simulink model "gmStateSpaceHDL_buck_convert_test1_REFERENCE"  (R2025a)
settings: Solver=FixedStepDiscrete  StartTime=0.0  StopTime=0.005  RelTol=1e-3  AbsTol=1e-3
InitFcn:
  | load('C:\Users\bensa\Desktop\PI3_FPGA_BuckConverter\sschdl\buck_convert_test1\stateSpaceParameters.mat');
model workspace (MAT data in the model file):
  NoaFutureIOMap{1}.PortName = 'rst'
  NoaFutureIOMap{1}.PortType = 'Inport'
  NoaFutureIOMap{1}.DataType = 'uint32'
  NoaFutureIOMap{1}.IOInterface = 'AXI4-Lite'
  NoaFutureIOMap{1}.IOInterfaceMapping = 'x"100"'
  NoaFutureIOMap{2}.PortName = 'duty'
  NoaFutureIOMap{2}.PortType = 'Inport'
  NoaFutureIOMap{2}.DataType = 'uint32'
  NoaFutureIOMap{2}.IOInterface = 'AXI4-Lite'
  NoaFutureIOMap{2}.IOInterfaceMapping = 'x"104"'
  NoaFutureIOMap{3}.PortName = 'freq'
  NoaFutureIOMap{3}.PortType = 'Inport'
  NoaFutureIOMap{3}.DataType = 'uint32'
  NoaFutureIOMap{3}.IOInterface = 'AXI4-Lite'
  NoaFutureIOMap{3}.IOInterfaceMapping = 'x"108"'
  NoaFutureIOMap{4}.PortName = 'en'
  NoaFutureIOMap{4}.PortType = 'Inport'
  NoaFutureIOMap{4}.DataType = 'uint32'
  NoaFutureIOMap{4}.IOInterface = 'AXI4-Lite'
  NoaFutureIOMap{4}.IOInterfaceMapping = 'x"10C"'
  NoaFutureIOMap{5}.PortName = 'vout'
  NoaFutureIOMap{5}.PortType = 'Outport'
  NoaFutureIOMap{5}.DataType = 'single'
  NoaFutureIOMap{5}.IOInterface = 'DAQ Channel 0 [0:31]'
  NoaFutureIOMap{5}.IOInterfaceMapping = '[0:31]'
  NoaFutureIOMap{6}.PortName = 'vin'
  NoaFutureIOMap{6}.PortType = 'Outport'
  NoaFutureIOMap{6}.DataType = 'single'
  NoaFutureIOMap{6}.IOInterface = 'DAQ Channel 1 [0:31]'
  NoaFutureIOMap{6}.IOInterfaceMapping = '[0:31]'
  NoaFutureIOMap{7}.PortName = 'vout_a'
  NoaFutureIOMap{7}.PortType = 'Outport'
  NoaFutureIOMap{7}.DataType = 'sfix32_En27'
  NoaFutureIOMap{7}.IOInterface = 'Analog Output 0 [0:31]'
  NoaFutureIOMap{7}.IOInterfaceMapping = '[0:31]'
  NoaFutureIOMap{7}.NoaBlockParameters.SignalMin = '0'
  NoaFutureIOMap{7}.NoaBlockParameters.SignalMax = '12'
  NoaFutureIOMap{7}.NoaBlockParameters.VoltageMin = '0'
  NoaFutureIOMap{7}.NoaBlockParameters.VoltageMax = '4'
  NoaFutureIOMap{7}.NoaBlockParameters.LUT_Signals = '[0          1.2          2.4          3.6          4.8            6          7.2          8.4          9.6         10.8           12]'
  NoaFutureIOMap{7}.NoaBlockParameters.LUT_Values = '[0         0.4         0.8         1.2         1.6           2         2.4         2.8         3.2         3.6           4]'
values from neighbouring files (symbols this model uses):
  stateSpaceParameters_1 =     [stateSpaceParameters.mat]
libraries: hdlsllib x4, hdlssclib x4, library_AnalogOut x1, simulink x1
CloseFcn:
  | clear stateSpaceParameters_1
settings Model: DataTypeOverride=Off  Creator=bensa  LastModifiedBy=bensa
settings SolverCC: AutoScaleAbsTol=off  AlgebraicLoopSolver=TrustRegion  MaxZcPerStep=1.0
settings OptimizationCC: BlockReduction=off  ConditionallyExecuteInputs=off  DefaultParameterBehavior=Inlined  InheritOutputTypeSmallerThanSingle=on
settings DebuggingCC: AlgebraicLoopMsg=error  ArtificialAlgebraicLoopMsg=error  SingleTaskRateTransMsg=error  UnconnectedInputMsg=warning  UnconnectedOutputMsg=warning  UnconnectedLineMsg=warning  SymbolicDimsDataTypeCodeGenerationDiagnostic=none
settings HardwareCC: ProdBitPerPointer=32.0  ProdBitPerSizeT=32.0  ProdBitPerPtrDiffT=32.0  ProdLargestAtomicFloat=None  ProdIntDivRoundTo=Undefined  ProdEndianess=Unspecified  ProdWordSize=32.0  ProdHWDeviceType=ASIC/FPGA->ASIC/FPGA  TargetBitPerPointer=64.0  TargetBitPerSizeT=64.0  TargetBitPerPtrDiffT=64.0  TargetLongLongMode=on  TargetIntDivRoundTo=Zero  TargetEndianess=LittleEndian  TargetWordSize=64.0  TargetHWDeviceType=Custom Processor->MATLAB Host Computer  ProdEqTarget=off
settings ModelReferenceCC: EnableRefExpFcnMdlSchedulingChecks=on
settings SFSimCC: CustomCodeUndefinedFunction=UseInterfaceOnly
settings RTWCC: GPUComputeCapability=3.5  DLArmComputeVersion=19.05
settings SimscapeCC: SimscapeLogType=all  SimscapeLogSimulationStatistics=on  SimscapeLogDataHistory=10000.0

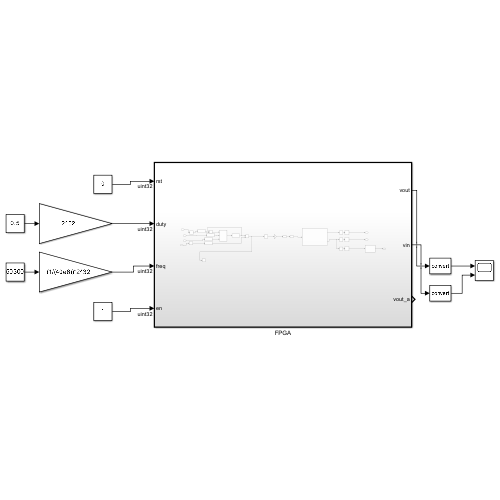
[thumbnail: Simulink's stored preview of the top-level diagram]
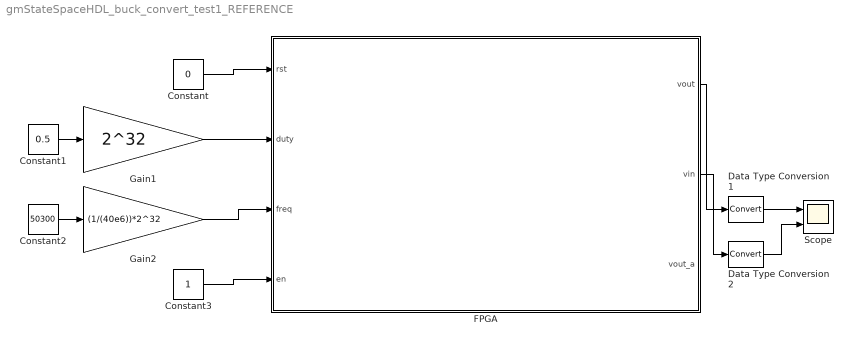
== system gmStateSpaceHDL_buck_convert_test1_REFERENCE ==
  Constant : Constant  Value=0  OutDataTypeStr=uint32  SampleTime=25e-9
  Constant1 : Constant  Value=0.5  OutDataTypeStr=double  SampleTime=25e-9
  Constant2 : Constant  Value=50300  SampleTime=25e-9
  Constant3 : Constant  OutDataTypeStr=uint32  SampleTime=25e-9
  Data Type Conversion1 : DataTypeConversion  RndMeth=Nearest  SaturateOnIntegerOverflow=off  LockScale=on
  Data Type Conversion2 : DataTypeConversion  RndMeth=Nearest  SaturateOnIntegerOverflow=off  LockScale=on
  FPGA : Subsystem  TreatAsAtomicUnit=on
  Gain1 : Gain  Gain=2^32  OutDataTypeStr=uint32
  Gain2 : Gain  Gain=(1/(40e6))*2^32  OutDataTypeStr=uint32
  Scope : Scope  NumInputPorts=2
      settings: ActiveDisplayYMinimum=-1.4999999999999996  ActiveDisplayYMaximum=13.5
  wires:
  Data Type Conversion1/1 -> Scope/1
  Data Type Conversion2/1 -> Scope/2
  FPGA/1(vout) -> Data Type Conversion1/1
  FPGA/2(vin) -> Data Type Conversion2/1
  Constant1/1 -> Gain1/1
  Constant/1 -> FPGA/1(rst)
  Constant2/1 -> Gain2/1
  Gain1/1 -> FPGA/2(duty)
  Gain2/1 -> FPGA/3(freq)
  Constant3/1 -> FPGA/4(en)

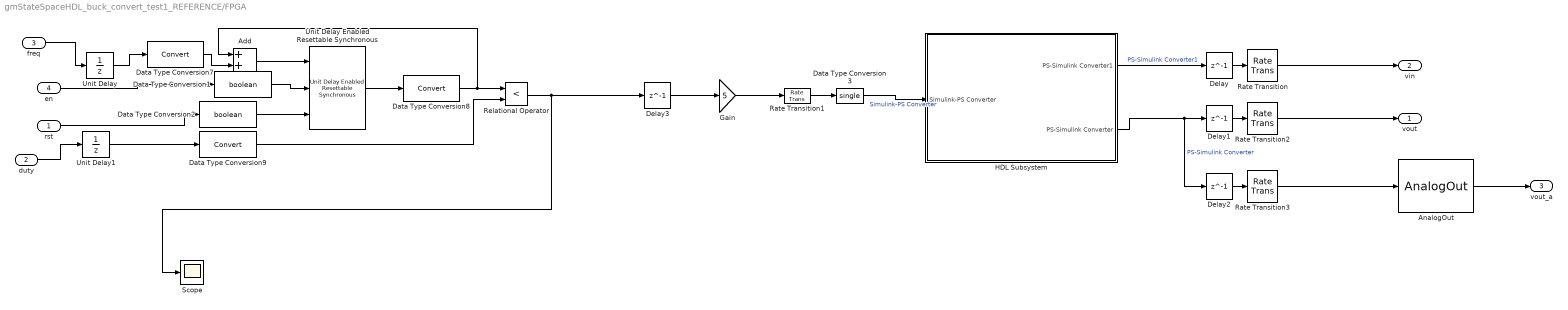
== system gmStateSpaceHDL_buck_convert_test1_REFERENCE/FPGA ==
  rst : Inport  OutDataTypeStr=uint32
  duty : Inport  Port=2  OutDataTypeStr=uint32
  freq : Inport  Port=3  OutDataTypeStr=uint32
  en : Inport  Port=4  OutDataTypeStr=uint32
  Add : Sum  OutDataTypeStr=uint32  AccumDataTypeStr=uint32
  AnalogOut : library_AnalogOut/AnalogOut  SignalMin=0  SignalMax=12  VoltageMin=0  VoltageMax=4
  Data Type Conversion1 : DataTypeConversion  OutDataTypeStr=boolean  SaturateOnIntegerOverflow=off  RndMeth=Floor
  Data Type Conversion2 : DataTypeConversion  OutDataTypeStr=boolean  SaturateOnIntegerOverflow=off  RndMeth=Floor
  Data Type Conversion3 : DataTypeConversion  OutDataTypeStr=single  RndMeth=Nearest  SaturateOnIntegerOverflow=off
  Data Type Conversion7 : DataTypeConversion  SaturateOnIntegerOverflow=off  RndMeth=Floor
  Data Type Conversion8 : DataTypeConversion  SaturateOnIntegerOverflow=off  RndMeth=Floor
  Data Type Conversion9 : DataTypeConversion  SaturateOnIntegerOverflow=off  RndMeth=Floor
  Delay{,1..3} (4 alike) : Delay  DelayLength=1
  Gain : Gain  Gain=5
  HDL Subsystem : Subsystem
  Rate Transition : RateTransition  OutPortSampleTime=25e-9
  Rate Transition1 : RateTransition  OutPortSampleTime=5e-08
  Rate Transition2 : RateTransition  OutPortSampleTime=25e-9
  Rate Transition3 : RateTransition  OutPortSampleTime=25e-9
  Relational Operator : RelationalOperator  Operator=<  OutDataTypeStr=boolean  RndMeth=Simplest  InputSameDT=off
  Scope : Scope
      settings: ActiveDisplayYMinimum=0.63603790546315564  ActiveDisplayYMaximum=1.1529609907534577
  Unit Delay : UnitDelay  SampleTime=-1  HasFrameUpgradeWarning=on
  Unit Delay Enabled Resettable Synchronous : hdlsllib/Discrete/Unit Delay Enabled Resettable Synchronous  InitialCondition=0.0  SampleTime=-1
  Unit Delay1 : UnitDelay  SampleTime=-1  HasFrameUpgradeWarning=on
  vout : Outport
  vin : Outport  Port=2
  vout_a : Outport  Port=3
  wires:
  HDL Subsystem/2(PS-Simulink Converter) -> Delay2/1, Delay1/1  "PS-Simulink Converter"
  HDL Subsystem/1(PS-Simulink Converter1) -> Delay/1  "PS-Simulink Converter1"
  Rate Transition1/1 -> Data Type Conversion3/1
  Data Type Conversion3/1 -> HDL Subsystem/1(Simulink-PS Converter)  "Simulink-PS Converter"
  Data Type Conversion8/1 -> Add/1, Relational Operator/1
  Add/1 -> Unit Delay Enabled Resettable Synchronous/1
  Unit Delay Enabled Resettable Synchronous/1 -> Data Type Conversion8/1
  Data Type Conversion7/1 -> Add/2
  Data Type Conversion9/1 -> Relational Operator/2
  Unit Delay1/1 -> Data Type Conversion9/1
  Unit Delay/1 -> Data Type Conversion7/1
  Relational Operator/1 -> Scope/1, Delay3/1
  freq/1 -> Unit Delay/1
  duty/1 -> Unit Delay1/1
  rst/1 -> Data Type Conversion2/1
  en/1 -> Data Type Conversion1/1
  Rate Transition/1 -> vin/1
  Rate Transition2/1 -> vout/1
  Delay/1 -> Rate Transition/1
  Delay1/1 -> Rate Transition2/1
  Delay2/1 -> Rate Transition3/1
  Rate Transition3/1 -> AnalogOut/1
  AnalogOut/1 -> vout_a/1
  Data Type Conversion1/1 -> Unit Delay Enabled Resettable Synchronous/2
  Data Type Conversion2/1 -> Unit Delay Enabled Resettable Synchronous/3
  Delay3/1 -> Gain/1
  Gain/1 -> Rate Transition1/1

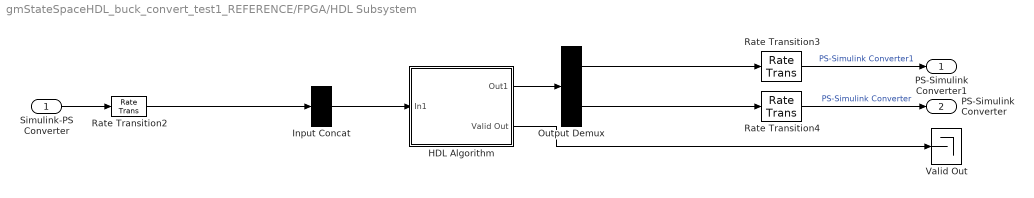
== system gmStateSpaceHDL_buck_convert_test1_REFERENCE/FPGA/HDL Subsystem ==
  Simulink-PS Converter : Inport
  HDL Algorithm : Subsystem
  Input Concat : Concatenate  NumInputs=1
  Output Demux : Demux  Outputs=2
  Rate Transition2 : RateTransition  Integrity=off  OutPortSampleTimeOpt=Multiple of input port sample time  OutPortSampleTimeMultiple=1/2
  Rate Transition3 : RateTransition  OutPortSampleTimeOpt=Multiple of input port sample time  OutPortSampleTimeMultiple=2
  Rate Transition4 : RateTransition  OutPortSampleTimeOpt=Multiple of input port sample time  OutPortSampleTimeMultiple=2
  Valid Out : Terminator
  PS-Simulink Converter1 : Outport
  PS-Simulink Converter : Outport  Port=2
  wires:
  Rate Transition3/1 -> PS-Simulink Converter1/1  "PS-Simulink Converter1"
  Rate Transition2/1 -> Input Concat/1
  HDL Algorithm/1(Out1) -> Output Demux/1
  Input Concat/1 -> HDL Algorithm/1(In1)
  Output Demux/2 -> Rate Transition4/1
  HDL Algorithm/2(Valid Out) -> Valid Out/1
  Output Demux/1 -> Rate Transition3/1
  Rate Transition4/1 -> PS-Simulink Converter/1  "PS-Simulink Converter"
  Simulink-PS Converter/1 -> Rate Transition2/1

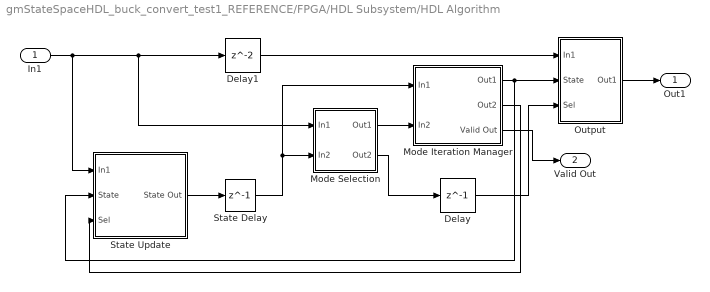
== system gmStateSpaceHDL_buck_convert_test1_REFERENCE/FPGA/HDL Subsystem/HDL Algorithm ==
  In1 : Inport
  Delay : Delay  DelayLength=1
  Delay1 : Delay
  Mode Iteration Manager : Subsystem
  Mode Selection : Subsystem
  Output : Subsystem
  State Delay : Delay  DelayLength=1  InitialCondition=single(stateSpaceParameters_1.X0)
  State Update : Subsystem
  Out1 : Outport  VectorParamsAs1DForOutWhenUnconnected=off
  Valid Out : Outport  Port=2  VectorParamsAs1DForOutWhenUnconnected=off
  wires:
  Mode Iteration Manager/2(Out2) -> State Update/3(Sel)
  In1/1 -> Mode Selection/1(In1), Delay1/1, State Update/1(In1)
  State Update/1(State Out) -> State Delay/1
  Mode Selection/1(Out1) -> Mode Iteration Manager/2(In2)
  Delay1/1 -> Output/1(In1)
  State Delay/1 -> Mode Iteration Manager/1(In1), Mode Selection/2(In2)
  Mode Selection/2(Out2) -> Delay/1
  Mode Iteration Manager/1(Out1) -> State Update/2(State), Output/2(State)
  Mode Iteration Manager/3(Valid Out) -> Valid Out/1
  Delay/1 -> Output/3(Sel)
  Output/1(Out1) -> Out1/1

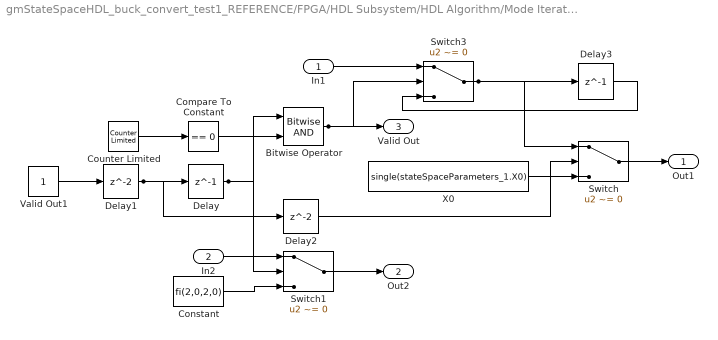
== system gmStateSpaceHDL_buck_convert_test1_REFERENCE/FPGA/HDL Subsystem/HDL Algorithm/Mode Iteration Manager ==
  In1 : Inport  LockScale=on
  In2 : Inport  Port=2  OutDataTypeStr=fixdt(0,2,0)  LockScale=on
  Bitwise Operator : simulink/Logic and Bit Operations/Bitwise Operator  logicop=AND  UseBitMask=off  NumInputPorts=2  BitMask=bin2dec('11011001')  BitMaskRealWorld=Stored Integer
      settings: LibrarySourceBlock=|
      | hdlsllib/Logic and Bit
      | Operations/Bitwise
      | Operator
  Compare To Constant : hdlsllib/Logic and Bit Operations/Compare To Constant  relop===  const=0  OutDataTypeStr=boolean
  Constant : Constant  Value=fi(2,0,2,0)  SampleTime=2.5e-08  LockScale=on
  Counter Limited : hdlsllib/Sources/Counter Limited  uplimit=1  tsamp=-1
  Delay : Delay  DelayLength=1
  Delay1 : Delay
  Delay2 : Delay
  Delay3 : Delay  DelayLength=1
  Switch : Switch  Criteria=u2 ~= 0  SaturateOnIntegerOverflow=off  InputSameDT=off
  Switch1 : Switch  Criteria=u2 ~= 0  SaturateOnIntegerOverflow=off  InputSameDT=off  OutDataTypeStr=Inherit: Same as first input
      settings: LockScale=on
  Switch3 : Switch  Criteria=u2 ~= 0  SaturateOnIntegerOverflow=off  InputSameDT=off
  Valid Out1 : Constant  OutDataTypeStr=boolean  SampleTime=2.5e-08
  X0 : Constant  Value=single(stateSpaceParameters_1.X0)  SampleTime=2.5e-08
  Out1 : Outport  OutDataTypeStr=single  VectorParamsAs1DForOutWhenUnconnected=off
  Out2 : Outport  Port=2  VectorParamsAs1DForOutWhenUnconnected=off
  Valid Out : Outport  Port=3  VectorParamsAs1DForOutWhenUnconnected=off
  wires:
  Constant/1 -> Switch1/3
  X0/1 -> Switch/3
  Valid Out1/1 -> Delay1/1
  Counter Limited/1 -> Compare To Constant/1
  In1/1 -> Switch3/1
  Delay/1 -> Switch1/2, Bitwise Operator/1
  Delay1/1 -> Delay2/1, Delay/1
  Compare To Constant/1 -> Bitwise Operator/2
  In2/1 -> Switch1/1
  Bitwise Operator/1 -> Switch3/2, Valid Out/1
  Delay2/1 -> Switch/2
  Switch1/1 -> Out2/1
  Switch3/1 -> Delay3/1, Switch/1
  Delay3/1 -> Switch3/3
  Switch/1 -> Out1/1

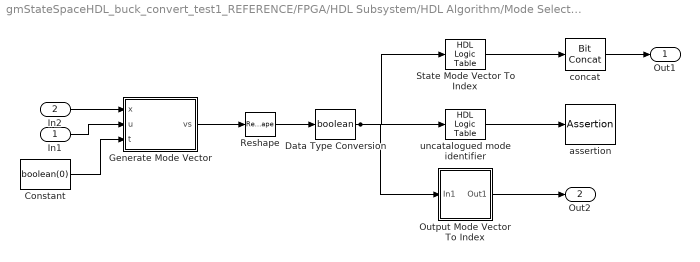
== system gmStateSpaceHDL_buck_convert_test1_REFERENCE/FPGA/HDL Subsystem/HDL Algorithm/Mode Selection ==
  In1 : Inport
  In2 : Inport  Port=2  LockScale=on
  Constant : Constant  Value=boolean(0)  SampleTime=2.5e-08
  Data Type Conversion : DataTypeConversion  OutDataTypeStr=boolean  RndMeth=Nearest  SaturateOnIntegerOverflow=off
  Generate Mode Vector : MATLAB Function  TreatAsAtomicUnit=on
  Output Mode Vector To Index : Subsystem
  Reshape : Reshape
  State Mode Vector To Index : hdlssclib/HDL Logic Table  InputTable=stateSpaceParameters_1.logicTableInput  OutputTable=stateSpaceParameters_1.logicTableOutput
  assertion : Assertion  StopWhenAssertionFail=off
  concat : hdlsllib/Logic and Bit Operations/Bit Concat  numInputs=1
  uncatalogued mode identifier : hdlssclib/HDL Logic Table  InputTable=stateSpaceParameters_1.logicTableInput  OutputTable=ones(size(stateSpaceParameters_1.logicTableOutput,1),1)
  Out1 : Outport  VectorParamsAs1DForOutWhenUnconnected=off  LockScale=on
  Out2 : Outport  Port=2  VectorParamsAs1DForOutWhenUnconnected=off
  wires:
  Data Type Conversion/1 -> State Mode Vector To Index/1, uncatalogued mode identifier/1, Output Mode Vector To Index/1(In1)
  In2/1 -> Generate Mode Vector/1(x)
  In1/1 -> Generate Mode Vector/2(u)
  Generate Mode Vector/1(vs) -> Reshape/1
  Constant/1 -> Generate Mode Vector/3(t)
  Reshape/1 -> Data Type Conversion/1
  concat/1 -> Out1/1
  State Mode Vector To Index/1 -> concat/1
  uncatalogued mode identifier/1 -> assertion/1
  Output Mode Vector To Index/1(Out1) -> Out2/1

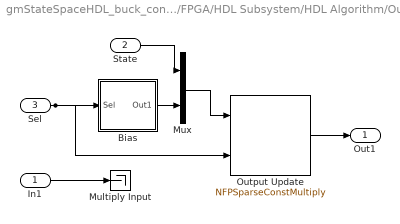
== system gmStateSpaceHDL_buck_convert_test1_REFERENCE/FPGA/HDL Subsystem/HDL Algorithm/Output ==
  In1 : Inport
  State : Inport  Port=2
  Sel : Inport  Port=3  LockScale=on
  Bias : Subsystem
  Multiply Input : Terminator
  Mux : Mux  Inputs=2
  Output Update : hdlssclib/NFPSparseConstMultiply  MatrixSource=Dialog  constMatrix=single([stateSpaceParameters_1.Cd repmat(eye(2),[1,1,1])])  MatrixType=single  MatrixSize=[1 1]  ColumnIndices=[1]  RowIndices=[1]  PropDataType=single  defWL=48
  Out1 : Outport  VectorParamsAs1DForOutWhenUnconnected=off
  wires:
  In1/1 -> Multiply Input/1
  Sel/1 -> Output Update/2, Bias/1(Sel)
  State/1 -> Mux/1
  Bias/1(Out1) -> Mux/2
  Mux/1 -> Output Update/1
  Output Update/1 -> Out1/1

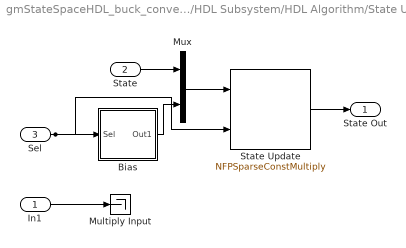
== system gmStateSpaceHDL_buck_convert_test1_REFERENCE/FPGA/HDL Subsystem/HDL Algorithm/State Update ==
  In1 : Inport
  State : Inport  Port=2
  Sel : Inport  Port=3  LockScale=on
  Bias : Subsystem
  Multiply Input : Terminator
  Mux : Mux  Inputs=2
  State Update : hdlssclib/NFPSparseConstMultiply  MatrixSource=Dialog  constMatrix=single([stateSpaceParameters_1.Ad repmat(eye(5),[1,1,4])])  MatrixType=single  MatrixSize=[1 1]  ColumnIndices=[1]  RowIndices=[1]  PropDataType=single  defWL=48
  State Out : Outport  OutDataTypeStr=single  VectorParamsAs1DForOutWhenUnconnected=off
  wires:
  Sel/1 -> State Update/2, Bias/1(Sel)
  State/1 -> Mux/1
  In1/1 -> Multiply Input/1
  Bias/1(Out1) -> Mux/2
  Mux/1 -> State Update/1
  State Update/1 -> State Out/1

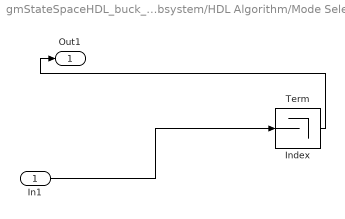
== system gmStateSpaceHDL_buck_convert_test1_REFERENCE/FPGA/HDL Subsystem/HDL Algorithm/Mode Selection/Output Mode Vector To Index ==
  In1 : Inport
  Index : Constant  Value=fi(0,0,1,0)  SampleTime=2.5e-08  LockScale=on
  Term : Terminator
  Out1 : Outport  VectorParamsAs1DForOutWhenUnconnected=off
  wires:
  In1/1 -> Term/1
  Index/1 -> Out1/1

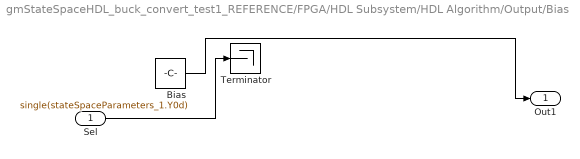
== system gmStateSpaceHDL_buck_convert_test1_REFERENCE/FPGA/HDL Subsystem/HDL Algorithm/Output/Bias ==
  Sel : Inport  LockScale=on
  Bias : Constant  Value=single(stateSpaceParameters_1.Y0d)  SampleTime=2.5e-08
  Terminator : Terminator
  Out1 : Outport  VectorParamsAs1DForOutWhenUnconnected=off
  wires:
  Sel/1 -> Terminator/1
  Bias/1 -> Out1/1

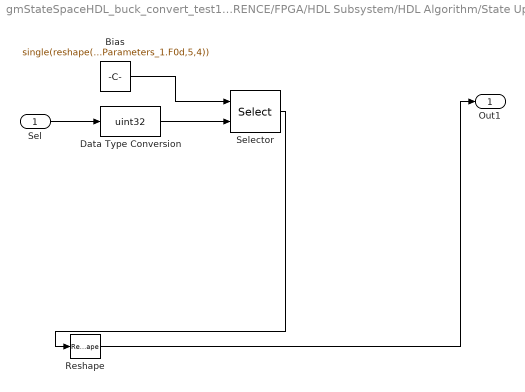
== system gmStateSpaceHDL_buck_convert_test1_REFERENCE/FPGA/HDL Subsystem/HDL Algorithm/State Update/Bias ==
  Sel : Inport  LockScale=on
  Bias : Constant  Value=single(reshape(stateSpaceParameters_1.F0d,5,4))  SampleTime=2.5e-08
  Data Type Conversion : DataTypeConversion  OutDataTypeStr=uint32  RndMeth=Nearest  SaturateOnIntegerOverflow=off
  Reshape : Reshape
  Selector : Selector  NumberOfDimensions=2  IndexMode=Zero-based  InputPortWidth=3  IndexOptions=Select all,Index vector (port)  Indices=[1 3]  OutputSizes=1
  Out1 : Outport  VectorParamsAs1DForOutWhenUnconnected=off
  wires:
  Selector/1 -> Reshape/1
  Bias/1 -> Selector/1
  Sel/1 -> Data Type Conversion/1
  Data Type Conversion/1 -> Selector/2
  Reshape/1 -> Out1/1

== matlab function gmStateSpaceHDL_buck_convert_test1_REFERENCE/FPGA/HDL Subsystem/HDL Algorithm/Mode Selection/Generate Mode Vector ==
  settings: fimath=fimath('RoundingMethod', 'Floor','OverflowAction', 'Wrap','ProductMode', 'FullPrecision', 'SumMode', 'FullPrecision')
  data: x input; u input; vs output; t input
function vs = compute_modes(x, u, t)

  tmp1 = ((-1.0) .* x(3));
  tmp2 = u(1);

  v1 = (tmp1 > (0.7));
  v2 = (tmp2 > (2.0));

  vs = [v1 v2];

end
